simulink model "MHILSimTDFixpoint"  (R2021b)
settings: Solver=VariableStepAuto  StartTime=0.0  StopTime=10.0  RelTol=1e-3
values from neighbouring files (symbols this model uses):
  m = tddbl_model    [HILSimModel.m]
libraries: simulink x54
(part 2 of 2)

== system MHILSimTDFixpoint/slice_1/u_nlf ==
  x : Inport
  Add : Sum  OutDataTypeStr=uint64
  Add1 : Sum  OutDataTypeStr=m.datatype.slice
  Add2 : Sum  Inputs=+-  OutDataTypeStr=m.datatype.slice
  Bitwise Operator : simulink/Logic and Bit Operations/Bitwise Operator  logicop=AND  UseBitMask=on  BitMask=bitxor((bitsll(1,m.datatype.slice_sz)-1), bitsll(1,m.datatype.slice_sz - m.datatype.nlf_lut_addr_sz)-1)  BitMaskRealWorld=Stored Integer
  Bitwise Operator1 : simulink/Logic and Bit Operations/Bitwise Operator  logicop=AND  UseBitMask=on  BitMask=bitsll(1,m.datatype.slice_sz - m.datatype.nlf_lut_addr_sz)-1  BitMaskRealWorld=Stored Integer
  Bitwise Operator2 : simulink/Logic and Bit Operations/Bitwise Operator  logicop=AND  UseBitMask=on  BitMask=bitsll(1,m.datatype.nlf_lut_addr_sz)-1  BitMaskRealWorld=Stored Integer
  Constant : Constant  OutDataTypeStr=uint64
  Constant1 : Constant  OutDataTypeStr=m.datatype.const
  Data Type Conversion1 : DataTypeConversion  OutDataTypeStr=int64  ConvertRealWorld=Stored Integer (SI)
  Data Type Conversion2 : DataTypeConversion  OutDataTypeStr=fixdt(0,m.datatype.slice_sz - m.datatype.nlf_lut_addr_sz,m.datatype.slice_sz - m.datatype.nlf_lut_addr_sz)  ConvertRealWorld=Stored Integer (SI)
  Data Type Conversion3 : DataTypeConversion  OutDataTypeStr=m.datatype.slice
  Direct Lookup Table (n-D) : LookupNDDirect  NumberOfTableDimensions=1  Table=m.slice1.u_nlf.lut  TableDataTypeStr=m.datatype.nlf
  Direct Lookup Table (n-D)1 : LookupNDDirect  NumberOfTableDimensions=1  Table=m.slice1.u_nlf.lut  TableDataTypeStr=m.datatype.nlf
  Gain : Gain  Gain=m.slice1.u_nlf.presc  OutDataTypeStr=fixdt(1,m.datatype.slice_sz,m.datatype.slice_sz-1)
  Gain1 : Gain  Gain=1/(2^(m.datatype.slice_sz - m.datatype.nlf_lut_addr_sz))  OutDataTypeStr=uint64
  Gain2 : Gain  Gain=m.slice1.u_nlf.gain  OutDataTypeStr=m.datatype.slice
  Product : Product  OutDataTypeStr=m.datatype.slice
  Product1 : Product  OutDataTypeStr=m.datatype.slice
  f(x) : Outport
  wires:
  Direct Lookup Table (n-D)/1 -> Product/1
  Data Type Conversion2/1 -> Data Type Conversion3/1
  Product1/1 -> Add1/2
  Direct Lookup Table (n-D)1/1 -> Product1/1
  Bitwise Operator/1 -> Gain1/1
  Add2/1 -> Product/2
  Gain1/1 -> Add/1, Direct Lookup Table (n-D)/1
  Gain/1 -> Data Type Conversion1/1
  Data Type Conversion3/1 -> Product1/2, Add2/2
  Data Type Conversion1/1 -> Bitwise Operator1/1, Bitwise Operator/1
  Add1/1 -> Gain2/1
  Constant1/1 -> Add2/1
  Constant/1 -> Add/2
  Product/1 -> Add1/1
  Bitwise Operator1/1 -> Data Type Conversion2/1
  Add/1 -> Bitwise Operator2/1
  x/1 -> Gain/1
  Gain2/1 -> f(x)/1
  Bitwise Operator2/1 -> Direct Lookup Table (n-D)1/1

== system MHILSimTDFixpoint/slice_1/x_nlf ==
  x : Inport
  Add : Sum  OutDataTypeStr=uint64
  Add1 : Sum  OutDataTypeStr=m.datatype.slice
  Add2 : Sum  Inputs=+-  OutDataTypeStr=m.datatype.slice
  Bitwise Operator : simulink/Logic and Bit Operations/Bitwise Operator  logicop=AND  UseBitMask=on  BitMask=bitxor((bitsll(1,m.datatype.slice_sz)-1), bitsll(1,m.datatype.slice_sz - m.datatype.nlf_lut_addr_sz)-1)  BitMaskRealWorld=Stored Integer
  Bitwise Operator1 : simulink/Logic and Bit Operations/Bitwise Operator  logicop=AND  UseBitMask=on  BitMask=bitsll(1,m.datatype.slice_sz - m.datatype.nlf_lut_addr_sz)-1  BitMaskRealWorld=Stored Integer
  Bitwise Operator2 : simulink/Logic and Bit Operations/Bitwise Operator  logicop=AND  UseBitMask=on  BitMask=bitsll(1,m.datatype.nlf_lut_addr_sz)-1  BitMaskRealWorld=Stored Integer
  Constant : Constant  OutDataTypeStr=uint64
  Constant1 : Constant  OutDataTypeStr=m.datatype.const
  Data Type Conversion1 : DataTypeConversion  OutDataTypeStr=int64  ConvertRealWorld=Stored Integer (SI)
  Data Type Conversion2 : DataTypeConversion  OutDataTypeStr=fixdt(0,m.datatype.slice_sz - m.datatype.nlf_lut_addr_sz,m.datatype.slice_sz - m.datatype.nlf_lut_addr_sz)  ConvertRealWorld=Stored Integer (SI)
  Data Type Conversion3 : DataTypeConversion  OutDataTypeStr=m.datatype.slice
  Direct Lookup Table (n-D) : LookupNDDirect  NumberOfTableDimensions=1  Table=m.slice1.x_nlf.lut  TableDataTypeStr=m.datatype.nlf
  Direct Lookup Table (n-D)1 : LookupNDDirect  NumberOfTableDimensions=1  Table=m.slice1.x_nlf.lut  TableDataTypeStr=m.datatype.nlf
  Gain : Gain  Gain=m.slice1.x_nlf.presc  OutDataTypeStr=fixdt(1,m.datatype.slice_sz,m.datatype.slice_sz-1)
  Gain1 : Gain  Gain=1/(2^(m.datatype.slice_sz - m.datatype.nlf_lut_addr_sz))  OutDataTypeStr=uint64
  Gain2 : Gain  Gain=m.slice1.x_nlf.gain  OutDataTypeStr=m.datatype.slice
  Product : Product  OutDataTypeStr=m.datatype.slice
  Product1 : Product  OutDataTypeStr=m.datatype.slice
  f(x) : Outport
  wires:
  Direct Lookup Table (n-D)/1 -> Product/1
  Data Type Conversion2/1 -> Data Type Conversion3/1
  Product1/1 -> Add1/2
  Direct Lookup Table (n-D)1/1 -> Product1/1
  Bitwise Operator/1 -> Gain1/1
  Add2/1 -> Product/2
  Gain1/1 -> Add/1, Direct Lookup Table (n-D)/1
  Gain/1 -> Data Type Conversion1/1
  Data Type Conversion3/1 -> Product1/2, Add2/2
  Data Type Conversion1/1 -> Bitwise Operator1/1, Bitwise Operator/1
  Add1/1 -> Gain2/1
  Constant1/1 -> Add2/1
  Constant/1 -> Add/2
  Product/1 -> Add1/1
  Bitwise Operator1/1 -> Data Type Conversion2/1
  Add/1 -> Bitwise Operator2/1
  x/1 -> Gain/1
  Gain2/1 -> f(x)/1
  Bitwise Operator2/1 -> Direct Lookup Table (n-D)1/1

== system MHILSimTDFixpoint/slice_1/xdot_nlf ==
  x : Inport
  Add : Sum  OutDataTypeStr=uint64
  Add1 : Sum  OutDataTypeStr=m.datatype.slice
  Add2 : Sum  Inputs=+-  OutDataTypeStr=m.datatype.slice
  Bitwise Operator : simulink/Logic and Bit Operations/Bitwise Operator  logicop=AND  UseBitMask=on  BitMask=bitxor((bitsll(1,m.datatype.slice_sz)-1), bitsll(1,m.datatype.slice_sz - m.datatype.nlf_lut_addr_sz)-1)  BitMaskRealWorld=Stored Integer
  Bitwise Operator1 : simulink/Logic and Bit Operations/Bitwise Operator  logicop=AND  UseBitMask=on  BitMask=bitsll(1,m.datatype.slice_sz - m.datatype.nlf_lut_addr_sz)-1  BitMaskRealWorld=Stored Integer
  Bitwise Operator2 : simulink/Logic and Bit Operations/Bitwise Operator  logicop=AND  UseBitMask=on  BitMask=bitsll(1,m.datatype.nlf_lut_addr_sz)-1  BitMaskRealWorld=Stored Integer
  Constant : Constant  OutDataTypeStr=uint64
  Constant1 : Constant  OutDataTypeStr=m.datatype.const
  Data Type Conversion1 : DataTypeConversion  OutDataTypeStr=int64  ConvertRealWorld=Stored Integer (SI)
  Data Type Conversion2 : DataTypeConversion  OutDataTypeStr=fixdt(0,m.datatype.slice_sz - m.datatype.nlf_lut_addr_sz,m.datatype.slice_sz - m.datatype.nlf_lut_addr_sz)  ConvertRealWorld=Stored Integer (SI)
  Data Type Conversion3 : DataTypeConversion  OutDataTypeStr=m.datatype.slice
  Direct Lookup Table (n-D) : LookupNDDirect  NumberOfTableDimensions=1  Table=m.slice1.xd_nlf.lut  TableDataTypeStr=m.datatype.nlf
  Direct Lookup Table (n-D)1 : LookupNDDirect  NumberOfTableDimensions=1  Table=m.slice1.xd_nlf.lut  TableDataTypeStr=m.datatype.nlf
  Gain : Gain  Gain=m.slice1.xd_nlf.presc  OutDataTypeStr=fixdt(1,m.datatype.slice_sz,m.datatype.slice_sz-1)
  Gain1 : Gain  Gain=1/(2^(m.datatype.slice_sz - m.datatype.nlf_lut_addr_sz))  OutDataTypeStr=uint64
  Gain2 : Gain  Gain=m.slice1.xd_nlf.gain  OutDataTypeStr=m.datatype.slice
  Product : Product  OutDataTypeStr=m.datatype.slice
  Product1 : Product  OutDataTypeStr=m.datatype.slice
  f(x) : Outport
  wires:
  Direct Lookup Table (n-D)/1 -> Product/1
  Data Type Conversion2/1 -> Data Type Conversion3/1
  Product1/1 -> Add1/2
  Direct Lookup Table (n-D)1/1 -> Product1/1
  Bitwise Operator/1 -> Gain1/1
  Add2/1 -> Product/2
  Gain1/1 -> Add/1, Direct Lookup Table (n-D)/1
  Gain/1 -> Data Type Conversion1/1
  Data Type Conversion3/1 -> Product1/2, Add2/2
  Data Type Conversion1/1 -> Bitwise Operator1/1, Bitwise Operator/1
  Add1/1 -> Gain2/1
  Constant1/1 -> Add2/1
  Constant/1 -> Add/2
  Product/1 -> Add1/1
  Bitwise Operator1/1 -> Data Type Conversion2/1
  Add/1 -> Bitwise Operator2/1
  x/1 -> Gain/1
  Gain2/1 -> f(x)/1
  Bitwise Operator2/1 -> Direct Lookup Table (n-D)1/1

== system MHILSimTDFixpoint/slice_1/xdot_presc ==
  in : Inport
  cast_to_fp_slice : DataTypeConversion  OutDataTypeStr=m.datatype.slice
  mul_presc : Gain  Gain=m.slice1.xd_presc_mul  OutDataTypeStr=m.datatype.slice
  shift_presc : Gain  Gain=2^(-m.slice1.xd_presc_bitshift)  ParamDataTypeStr=uint64  OutDataTypeStr=m.datatype.accum
  out : Outport
  wires:
  in/1 -> shift_presc/1
  cast_to_fp_slice/1 -> mul_presc/1
  shift_presc/1 -> cast_to_fp_slice/1
  mul_presc/1 -> out/1

== system MHILSimTDFixpoint/slice_1/xdot_presc1 ==
  in : Inport
  cast_to_fp_slice : DataTypeConversion  OutDataTypeStr=m.datatype.slice
  mul_presc : Gain  Gain=m.slice1.x_presc_mul  OutDataTypeStr=m.datatype.slice
  shift_presc : Gain  Gain=2^(-m.slice1.x_presc_bitshift)  ParamDataTypeStr=uint64  OutDataTypeStr=m.datatype.accum
  out : Outport
  wires:
  in/1 -> shift_presc/1
  cast_to_fp_slice/1 -> mul_presc/1
  shift_presc/1 -> cast_to_fp_slice/1
  mul_presc/1 -> out/1

== system MHILSimTDFixpoint/slice_2/int_xddot_xdot ==
  fdot : Inport
  Add : Sum  OutDataTypeStr=m.datatype.accum
  Add1 : Sum  Inputs=+-  OutDataTypeStr=m.datatype.slice
  Add2 : Sum  OutDataTypeStr=m.datatype.slice
  Unit Delay : UnitDelay  SampleTime=m.t_s  HasFrameUpgradeWarning=on
  Unit Delay1 : UnitDelay  SampleTime=m.t_s  HasFrameUpgradeWarning=on
  fp_prepend_zeros : DataTypeConversion  OutDataTypeStr=fixdt(1,m.datatype.slice_sz+m.int_scale_bits,m.datatype.slice_bin)
  fp_repr_shift_prescale : Gain  Gain=1/(2^m.int_scale_bits)  OutDataTypeStr=m.datatype.accum
  half : Gain  Gain=1/2  OutDataTypeStr=m.datatype.slice
  int_presc : Gain  Gain=m.int_dt_residual  OutDataTypeStr=m.datatype.slice
  f : Outport
  wires:
  int_presc/1 -> fp_prepend_zeros/1
  fp_repr_shift_prescale/1 -> Add/1
  Add/1 -> f/1, Unit Delay/1
  fp_prepend_zeros/1 -> fp_repr_shift_prescale/1
  Unit Delay/1 -> Add/2
  fdot/1 -> half/1, Add2/1
  Add1/1 -> int_presc/1
  Add2/1 -> Add1/1
  half/1 -> Add2/2, Unit Delay1/1
  Unit Delay1/1 -> Add1/2

== system MHILSimTDFixpoint/slice_2/int_xdot_x ==
  fdot : Inport
  Add : Sum  OutDataTypeStr=m.datatype.accum
  Add1 : Sum  OutDataTypeStr=m.datatype.slice
  Unit Delay : UnitDelay  SampleTime=m.t_s  HasFrameUpgradeWarning=on
  Unit Delay1 : UnitDelay  SampleTime=m.t_s  HasFrameUpgradeWarning=on
  fp_prepend_zeros : DataTypeConversion  OutDataTypeStr=fixdt(1,m.datatype.slice_sz+m.int_scale_bits,m.datatype.slice_bin)
  fp_repr_shift_prescale : Gain  Gain=1/(2^m.int_scale_bits)  OutDataTypeStr=m.datatype.accum
  half : Gain  Gain=1/2  OutDataTypeStr=m.datatype.slice
  int_presc : Gain  Gain=m.int_dt_residual  OutDataTypeStr=m.datatype.slice
  f : Outport
  wires:
  int_presc/1 -> fp_prepend_zeros/1
  fp_repr_shift_prescale/1 -> Add/1
  Add/1 -> f/1, Unit Delay/1
  fp_prepend_zeros/1 -> fp_repr_shift_prescale/1
  Unit Delay/1 -> Add/2
  fdot/1 -> Unit Delay1/1, Add1/1
  half/1 -> int_presc/1
  Add1/1 -> half/1
  Unit Delay1/1 -> Add1/2

== system MHILSimTDFixpoint/slice_2/u_nlf ==
  x : Inport
  Add : Sum  OutDataTypeStr=uint64
  Add1 : Sum  OutDataTypeStr=m.datatype.slice
  Add2 : Sum  Inputs=+-  OutDataTypeStr=m.datatype.slice
  Bitwise Operator : simulink/Logic and Bit Operations/Bitwise Operator  logicop=AND  UseBitMask=on  BitMask=bitxor((bitsll(1,m.datatype.slice_sz)-1), bitsll(1,m.datatype.slice_sz - m.datatype.nlf_lut_addr_sz)-1)  BitMaskRealWorld=Stored Integer
  Bitwise Operator1 : simulink/Logic and Bit Operations/Bitwise Operator  logicop=AND  UseBitMask=on  BitMask=bitsll(1,m.datatype.slice_sz - m.datatype.nlf_lut_addr_sz)-1  BitMaskRealWorld=Stored Integer
  Bitwise Operator2 : simulink/Logic and Bit Operations/Bitwise Operator  logicop=AND  UseBitMask=on  BitMask=bitsll(1,m.datatype.nlf_lut_addr_sz)-1  BitMaskRealWorld=Stored Integer
  Constant : Constant  OutDataTypeStr=uint64
  Constant1 : Constant  OutDataTypeStr=m.datatype.const
  Data Type Conversion1 : DataTypeConversion  OutDataTypeStr=int64  ConvertRealWorld=Stored Integer (SI)
  Data Type Conversion2 : DataTypeConversion  OutDataTypeStr=fixdt(0,m.datatype.slice_sz - m.datatype.nlf_lut_addr_sz,m.datatype.slice_sz - m.datatype.nlf_lut_addr_sz)  ConvertRealWorld=Stored Integer (SI)
  Data Type Conversion3 : DataTypeConversion  OutDataTypeStr=m.datatype.slice
  Direct Lookup Table (n-D) : LookupNDDirect  NumberOfTableDimensions=1  Table=m.slice2.u_nlf.lut  TableDataTypeStr=m.datatype.nlf
  Direct Lookup Table (n-D)1 : LookupNDDirect  NumberOfTableDimensions=1  Table=m.slice2.u_nlf.lut  TableDataTypeStr=m.datatype.nlf
  Gain : Gain  Gain=m.slice2.u_nlf.presc  OutDataTypeStr=fixdt(1,m.datatype.slice_sz,m.datatype.slice_sz-1)
  Gain1 : Gain  Gain=1/(2^(m.datatype.slice_sz - m.datatype.nlf_lut_addr_sz))  OutDataTypeStr=uint64
  Gain2 : Gain  Gain=m.slice2.u_nlf.gain  OutDataTypeStr=m.datatype.slice
  Product : Product  OutDataTypeStr=m.datatype.slice
  Product1 : Product  OutDataTypeStr=m.datatype.slice
  f(x) : Outport
  wires:
  Direct Lookup Table (n-D)/1 -> Product/1
  Data Type Conversion2/1 -> Data Type Conversion3/1
  Product1/1 -> Add1/2
  Direct Lookup Table (n-D)1/1 -> Product1/1
  Bitwise Operator/1 -> Gain1/1
  Add2/1 -> Product/2
  Gain1/1 -> Add/1, Direct Lookup Table (n-D)/1
  Gain/1 -> Data Type Conversion1/1
  Data Type Conversion3/1 -> Product1/2, Add2/2
  Data Type Conversion1/1 -> Bitwise Operator1/1, Bitwise Operator/1
  Add1/1 -> Gain2/1
  Constant1/1 -> Add2/1
  Constant/1 -> Add/2
  Product/1 -> Add1/1
  Bitwise Operator1/1 -> Data Type Conversion2/1
  Add/1 -> Bitwise Operator2/1
  x/1 -> Gain/1
  Gain2/1 -> f(x)/1
  Bitwise Operator2/1 -> Direct Lookup Table (n-D)1/1

== system MHILSimTDFixpoint/slice_2/x_nlf ==
  x : Inport
  Add : Sum  OutDataTypeStr=uint64
  Add1 : Sum  OutDataTypeStr=m.datatype.slice
  Add2 : Sum  Inputs=+-  OutDataTypeStr=m.datatype.slice
  Bitwise Operator : simulink/Logic and Bit Operations/Bitwise Operator  logicop=AND  UseBitMask=on  BitMask=bitxor((bitsll(1,m.datatype.slice_sz)-1), bitsll(1,m.datatype.slice_sz - m.datatype.nlf_lut_addr_sz)-1)  BitMaskRealWorld=Stored Integer
  Bitwise Operator1 : simulink/Logic and Bit Operations/Bitwise Operator  logicop=AND  UseBitMask=on  BitMask=bitsll(1,m.datatype.slice_sz - m.datatype.nlf_lut_addr_sz)-1  BitMaskRealWorld=Stored Integer
  Bitwise Operator2 : simulink/Logic and Bit Operations/Bitwise Operator  logicop=AND  UseBitMask=on  BitMask=bitsll(1,m.datatype.nlf_lut_addr_sz)-1  BitMaskRealWorld=Stored Integer
  Constant : Constant  OutDataTypeStr=uint64
  Constant1 : Constant  OutDataTypeStr=m.datatype.const
  Data Type Conversion1 : DataTypeConversion  OutDataTypeStr=int64  ConvertRealWorld=Stored Integer (SI)
  Data Type Conversion2 : DataTypeConversion  OutDataTypeStr=fixdt(0,m.datatype.slice_sz - m.datatype.nlf_lut_addr_sz,m.datatype.slice_sz - m.datatype.nlf_lut_addr_sz)  ConvertRealWorld=Stored Integer (SI)
  Data Type Conversion3 : DataTypeConversion  OutDataTypeStr=m.datatype.slice
  Direct Lookup Table (n-D) : LookupNDDirect  NumberOfTableDimensions=1  Table=m.slice2.x_nlf.lut  TableDataTypeStr=m.datatype.nlf
  Direct Lookup Table (n-D)1 : LookupNDDirect  NumberOfTableDimensions=1  Table=m.slice2.x_nlf.lut  TableDataTypeStr=m.datatype.nlf
  Gain : Gain  Gain=m.slice2.x_nlf.presc  OutDataTypeStr=fixdt(1,m.datatype.slice_sz,m.datatype.slice_sz-1)
  Gain1 : Gain  Gain=1/(2^(m.datatype.slice_sz - m.datatype.nlf_lut_addr_sz))  OutDataTypeStr=uint64
  Gain2 : Gain  Gain=m.slice2.x_nlf.gain  OutDataTypeStr=m.datatype.slice
  Product : Product  OutDataTypeStr=m.datatype.slice
  Product1 : Product  OutDataTypeStr=m.datatype.slice
  f(x) : Outport
  wires:
  Direct Lookup Table (n-D)/1 -> Product/1
  Data Type Conversion2/1 -> Data Type Conversion3/1
  Product1/1 -> Add1/2
  Direct Lookup Table (n-D)1/1 -> Product1/1
  Bitwise Operator/1 -> Gain1/1
  Add2/1 -> Product/2
  Gain1/1 -> Add/1, Direct Lookup Table (n-D)/1
  Gain/1 -> Data Type Conversion1/1
  Data Type Conversion3/1 -> Product1/2, Add2/2
  Data Type Conversion1/1 -> Bitwise Operator1/1, Bitwise Operator/1
  Add1/1 -> Gain2/1
  Constant1/1 -> Add2/1
  Constant/1 -> Add/2
  Product/1 -> Add1/1
  Bitwise Operator1/1 -> Data Type Conversion2/1
  Add/1 -> Bitwise Operator2/1
  x/1 -> Gain/1
  Gain2/1 -> f(x)/1
  Bitwise Operator2/1 -> Direct Lookup Table (n-D)1/1

== system MHILSimTDFixpoint/slice_2/xdot_nlf ==
  x : Inport
  Add : Sum  OutDataTypeStr=uint64
  Add1 : Sum  OutDataTypeStr=m.datatype.slice
  Add2 : Sum  Inputs=+-  OutDataTypeStr=m.datatype.slice
  Bitwise Operator : simulink/Logic and Bit Operations/Bitwise Operator  logicop=AND  UseBitMask=on  BitMask=bitxor((bitsll(1,m.datatype.slice_sz)-1), bitsll(1,m.datatype.slice_sz - m.datatype.nlf_lut_addr_sz)-1)  BitMaskRealWorld=Stored Integer
  Bitwise Operator1 : simulink/Logic and Bit Operations/Bitwise Operator  logicop=AND  UseBitMask=on  BitMask=bitsll(1,m.datatype.slice_sz - m.datatype.nlf_lut_addr_sz)-1  BitMaskRealWorld=Stored Integer
  Bitwise Operator2 : simulink/Logic and Bit Operations/Bitwise Operator  logicop=AND  UseBitMask=on  BitMask=bitsll(1,m.datatype.nlf_lut_addr_sz)-1  BitMaskRealWorld=Stored Integer
  Constant : Constant  OutDataTypeStr=uint64
  Constant1 : Constant  OutDataTypeStr=m.datatype.const
  Data Type Conversion1 : DataTypeConversion  OutDataTypeStr=int64  ConvertRealWorld=Stored Integer (SI)
  Data Type Conversion2 : DataTypeConversion  OutDataTypeStr=fixdt(0,m.datatype.slice_sz - m.datatype.nlf_lut_addr_sz,m.datatype.slice_sz - m.datatype.nlf_lut_addr_sz)  ConvertRealWorld=Stored Integer (SI)
  Data Type Conversion3 : DataTypeConversion  OutDataTypeStr=m.datatype.slice
  Direct Lookup Table (n-D) : LookupNDDirect  NumberOfTableDimensions=1  Table=m.slice2.xd_nlf.lut  TableDataTypeStr=m.datatype.nlf
  Direct Lookup Table (n-D)1 : LookupNDDirect  NumberOfTableDimensions=1  Table=m.slice2.xd_nlf.lut  TableDataTypeStr=m.datatype.nlf
  Gain : Gain  Gain=m.slice2.xd_nlf.presc  OutDataTypeStr=fixdt(1,m.datatype.slice_sz,m.datatype.slice_sz-1)
  Gain1 : Gain  Gain=1/(2^(m.datatype.slice_sz - m.datatype.nlf_lut_addr_sz))  OutDataTypeStr=uint64
  Gain2 : Gain  Gain=m.slice2.xd_nlf.gain  OutDataTypeStr=m.datatype.slice
  Product : Product  OutDataTypeStr=m.datatype.slice
  Product1 : Product  OutDataTypeStr=m.datatype.slice
  f(x) : Outport
  wires:
  Direct Lookup Table (n-D)/1 -> Product/1
  Data Type Conversion2/1 -> Data Type Conversion3/1
  Product1/1 -> Add1/2
  Direct Lookup Table (n-D)1/1 -> Product1/1
  Bitwise Operator/1 -> Gain1/1
  Add2/1 -> Product/2
  Gain1/1 -> Add/1, Direct Lookup Table (n-D)/1
  Gain/1 -> Data Type Conversion1/1
  Data Type Conversion3/1 -> Product1/2, Add2/2
  Data Type Conversion1/1 -> Bitwise Operator1/1, Bitwise Operator/1
  Add1/1 -> Gain2/1
  Constant1/1 -> Add2/1
  Constant/1 -> Add/2
  Product/1 -> Add1/1
  Bitwise Operator1/1 -> Data Type Conversion2/1
  Add/1 -> Bitwise Operator2/1
  x/1 -> Gain/1
  Gain2/1 -> f(x)/1
  Bitwise Operator2/1 -> Direct Lookup Table (n-D)1/1

== system MHILSimTDFixpoint/slice_2/xdot_presc ==
  in : Inport
  cast_to_fp_slice : DataTypeConversion  OutDataTypeStr=m.datatype.slice
  mul_presc : Gain  Gain=m.slice2.xd_presc_mul  OutDataTypeStr=m.datatype.slice
  shift_presc : Gain  Gain=2^(-m.slice2.xd_presc_bitshift)  ParamDataTypeStr=uint64  OutDataTypeStr=m.datatype.accum
  out : Outport
  wires:
  in/1 -> shift_presc/1
  cast_to_fp_slice/1 -> mul_presc/1
  shift_presc/1 -> cast_to_fp_slice/1
  mul_presc/1 -> out/1

== system MHILSimTDFixpoint/slice_2/xdot_presc1 ==
  in : Inport
  cast_to_fp_slice : DataTypeConversion  OutDataTypeStr=m.datatype.slice
  mul_presc : Gain  Gain=m.slice2.x_presc_mul  OutDataTypeStr=m.datatype.slice
  shift_presc : Gain  Gain=2^(-m.slice2.x_presc_bitshift)  ParamDataTypeStr=uint64  OutDataTypeStr=m.datatype.accum
  out : Outport
  wires:
  in/1 -> shift_presc/1
  cast_to_fp_slice/1 -> mul_presc/1
  shift_presc/1 -> cast_to_fp_slice/1
  mul_presc/1 -> out/1
